simulink model "Model"  (R2025b)
settings: Solver=VariableStepAuto  StartTime=0.0  StopTime=1  RelTol=1e-3
values from neighbouring files (symbols this model uses):
  g = 9.81    [Main.m]
  i0 = 0.0    (= 0)    [Main.m]    (also in anonimousFunction.m)
  i_stable = u_stable / R    [Main.m]
  M = 0.058    [Model_parameters.m]
  m = 0.058    [Main.m]    (also in anonimousFunction.m)
  R = 3.9924    [Main.m]    (also in Model_parameters.m = 2.8304; Resistance_ident.m = fitobject.p1; anonimousFunction.m = 2)
  v0 = 0    [Main.m]    (also in anonimousFunction.m)
  v_stable = 0    [Main.m]
  x0 = 0.02    [Main.m]    (also in anonimousFunction.m)
  x_stable = 0.01    [Main.m]
undefined symbols (not defined in the file or in its folder): K
settings Model: Creator=janis  LastModifiedBy=Tim

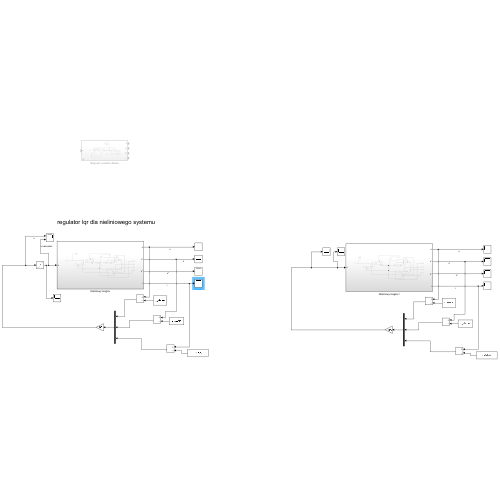
[thumbnail: Simulink's stored preview of the top-level diagram]
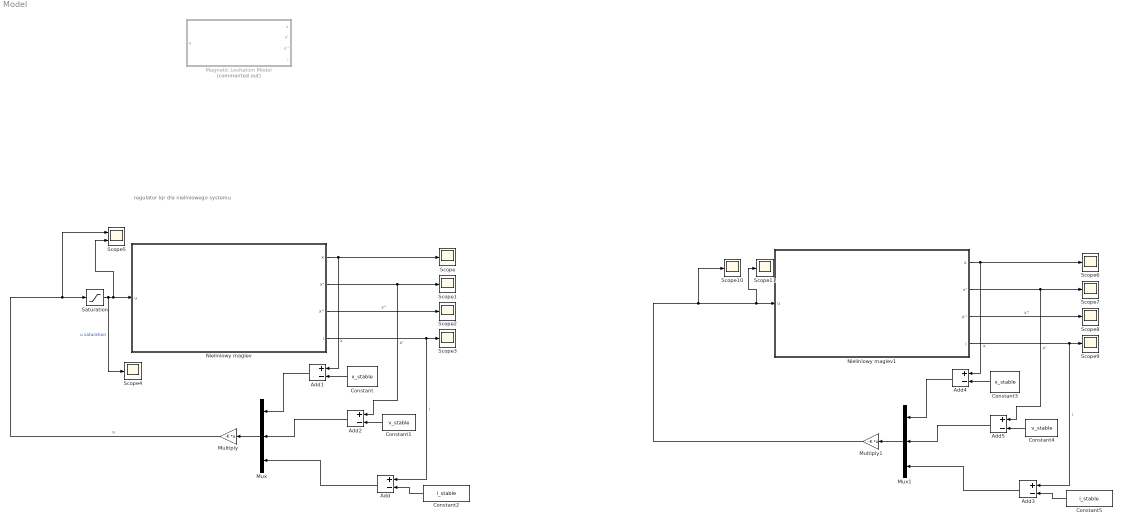
== system Model ==
  note: regulator lqr dla nieliniowego systemu
  Add{,1..5} (6 alike) : Sum  Inputs=+-
  Constant : Constant  Value=x_stable
  Constant1 : Constant  Value=v_stable
  Constant2 : Constant  Value=i_stable
  Constant3 : Constant  Value=x_stable
  Constant4 : Constant  Value=v_stable
  Constant5 : Constant  Value=i_stable
  Magnetic Levitation Model : Subsystem  Commented=on
  Multiply : Gain  Gain=-K  Multiplication=Matrix(K*u)
  Multiply1 : Gain  Gain=-K  Multiplication=Matrix(K*u)
  Mux : Mux  Inputs=3
  Mux1 : Mux  Inputs=3
  Nieliniowy maglev : Subsystem
  Nieliniowy maglev1 : Subsystem
  Saturation : Saturate  UpperLimit=11.3  LowerLimit=0
  Scope{,1..4,6..11} (11 alike) : Scope
      Scope settings: ActiveDisplayYMinimum=0.0081937181493075  ActiveDisplayYMaximum=0.026682726345841533  YLabel=x [m]
      Scope1 settings: ActiveDisplayYMinimum=-0.32675858583001738  ActiveDisplayYMaximum=0.19457434048931541  YLabel=x' [m/s]
      Scope10 settings: ActiveDisplayYMinimum=-8.0131796633081951  ActiveDisplayYMaximum=95.659493328647159  DataLoggingVariableName=ScopeData6
      Scope11 settings: ActiveDisplayYMinimum=-8.0131796633081951  ActiveDisplayYMaximum=95.659493328647159  DataLoggingVariableName=ScopeData7
      Scope2 settings: ActiveDisplayYMinimum=-15.369653428194885  ActiveDisplayYMaximum=12.607739269799431  YLabel=x'' [m/s^2]  DataLoggingVariableName=ScopeData2
      Scope3 settings: ActiveDisplayYMinimum=-0.53487282312330309  ActiveDisplayYMaximum=3.0849573402562789  YLabel=i [A]  DataLoggingVariableName=ScopeData3
      Scope4 settings: ActiveDisplayYMinimum=-0.37305316249219622  ActiveDisplayYMaximum=12.523736873656135  YLabel=u  DataLoggingVariableName=ScopeData4
      Scope6 settings: ActiveDisplayYMinimum=0.010968481395608059  ActiveDisplayYMaximum=0.021090683701156816  DataLoggingVariableName=ScopeData8
      Scope7 settings: ActiveDisplayYMinimum=-0.19832990389063207  ActiveDisplayYMaximum=0.16245757916094666  DataLoggingVariableName=ScopeData9
      Scope8 settings: ActiveDisplayYMinimum=-1  ActiveDisplayYMaximum=1  DataLoggingVariableName=ScopeData10
      Scope9 settings: ActiveDisplayYMinimum=-0.3151279377575355  ActiveDisplayYMaximum=2.83615143981782  DataLoggingVariableName=ScopeData11
  Scope5 : Scope  NumInputPorts=2
      settings: ActiveDisplayYMinimum=-56.44177745177619  ActiveDisplayYMaximum=512.64296076233984  DataLoggingVariableName=ScopeData5
  wires:
  Nieliniowy maglev/1(x) -> Scope/1, Add1/1  "x"
  Nieliniowy maglev/2(x') -> Add2/1, Scope1/1  "x'"
  Nieliniowy maglev/3(x'') -> Scope2/1  "x''"
  Nieliniowy maglev/4(i) -> Add/1, Scope3/1  "i"
  Constant2/1 -> Add/2
  Constant/1 -> Add1/2
  Constant1/1 -> Add2/2
  Mux/1 -> Multiply/1
  Add1/1 -> Mux/1
  Add2/1 -> Mux/2
  Multiply/1 -> Scope5/1, Saturation/1  "u"
  Add/1 -> Mux/3
  Saturation/1 -> Scope4/1, Scope5/2, Nieliniowy maglev/1(u)  "u saturation"
  Add3/1 -> Mux1/3
  Add4/1 -> Mux1/1
  Mux1/1 -> Multiply1/1
  Add5/1 -> Mux1/2
  Multiply1/1 -> Scope11/1, Nieliniowy maglev1/1(u), Scope10/1
  Nieliniowy maglev1/1(x) -> Scope6/1, Add4/1  "x"
  Constant3/1 -> Add4/2
  Nieliniowy maglev1/4(i) -> Add3/1, Scope9/1  "i"
  Nieliniowy maglev1/3(x'') -> Scope8/1  "x''"
  Nieliniowy maglev1/2(x') -> Add5/1, Scope7/1  "x'"
  Constant5/1 -> Add3/2
  Constant4/1 -> Add5/2

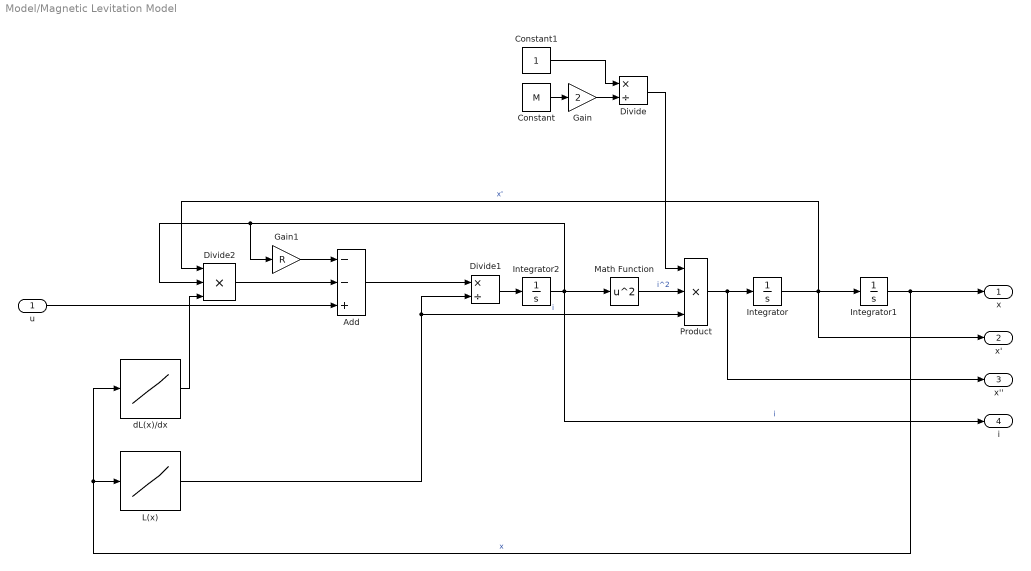
== system Model/Magnetic Levitation Model ==
  u : Inport
  Add : Sum  Inputs=--+
  Constant : Constant  Value=M
  Constant1 : Constant
  Divide : Product  Inputs=*/
  Divide1 : Product  Inputs=*/
  Divide2 : Product  Inputs=***
  Gain : Gain  Gain=2
  Gain1 : Gain  Gain=R
  Integrator : Integrator
  Integrator1 : Integrator
  Integrator2 : Integrator
  L(x) : Lookup_n-D  NumberOfTableDimensions=1  BreakpointsForDimension1=[-1:1]  Table=[-1:1]  InternalRulePriority=Speed  RndMeth=Simplest
  Math Function : Math  Operator=square
  Product : Product  Inputs=3
  dL(x)/dx : Lookup_n-D  NumberOfTableDimensions=1  BreakpointsForDimension1=[-1:1]  Table=[-1:1]  InternalRulePriority=Speed  RndMeth=Simplest
  x : Outport
  x' : Outport  Port=2
  x'' : Outport  Port=3
  i : Outport  Port=4
  wires:
  Gain1/1 -> Add/1
  L(x)/1 -> Divide1/2, Product/3  "i"
  Gain/1 -> Divide/2
  Divide2/1 -> Add/2
  Constant/1 -> Gain/1
  Integrator2/1 -> i/1, Gain1/1, Divide2/2, Math Function/1  "i"
  Integrator/1 -> x'/1, Divide2/1, Integrator1/1  "x'"
  Add/1 -> Divide1/1
  Integrator1/1 -> x/1, dL(x)/dx/1, L(x)/1  "x"
  Constant1/1 -> Divide/1
  Product/1 -> x''/1, Integrator/1
  Divide/1 -> Product/1
  Divide1/1 -> Integrator2/1
  dL(x)/dx/1 -> Divide2/3
  Math Function/1 -> Product/2  "i^2"
  u/1 -> Add/3

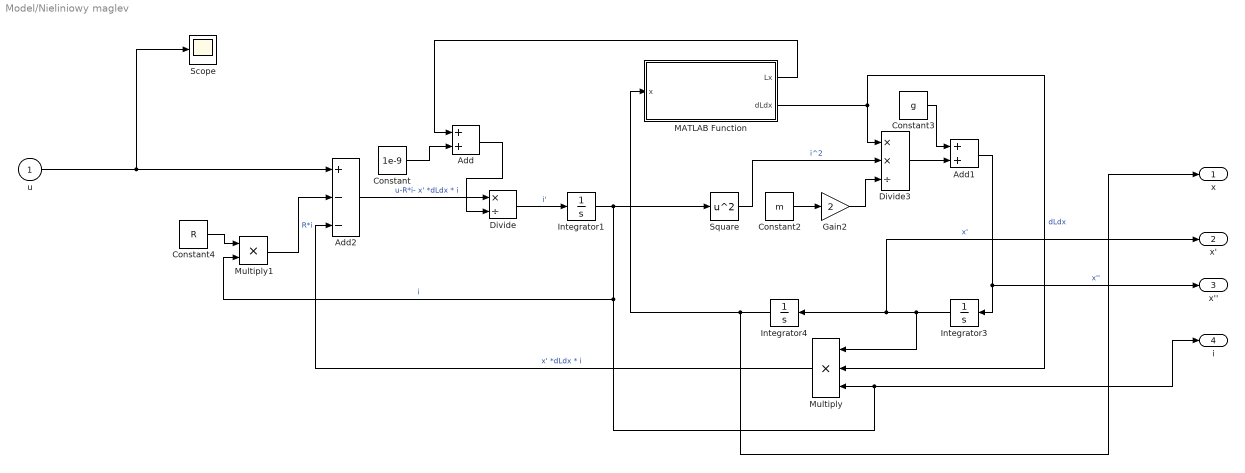
== system Model/Nieliniowy maglev ==
  u : Inport
  Add : Sum
  Add1 : Sum
  Add2 : Sum  Inputs=+--
  Constant : Constant  Value=1e-9
  Constant2 : Constant  Value=m
  Constant3 : Constant  Value=g
  Constant4 : Constant  Value=R
  Divide : Product  Inputs=*/
  Divide3 : Product  Inputs=**/
  Gain2 : Gain  Gain=2
  Integrator1 : Integrator  InitialCondition=i0
  Integrator3 : Integrator  InitialCondition=v0
  Integrator4 : Integrator  InitialCondition=x0
  MATLAB Function : MATLAB Function  TreatAsAtomicUnit=on
  Multiply : Product  Inputs=***
  Multiply1 : Product  Inputs=**
  Scope : Scope
      settings: ActiveDisplayYMinimum=-1  ActiveDisplayYMaximum=1  DataLoggingVariableName=ScopeData12
  Square : Math  Operator=square
  x : Outport
  x' : Outport  Port=2
  x'' : Outport  Port=3
  i : Outport  Port=4
  wires:
  Integrator3/1 -> Multiply/1, x'/1, Integrator4/1  "x'"
  Constant3/1 -> Add1/1
  MATLAB Function/2(dLdx) -> Divide3/1, Multiply/2  "dLdx"
  Add2/1 -> Divide/1  "u-R*i- x' *dLdx * i"
  Constant2/1 -> Gain2/1
  Integrator4/1 -> x/1, MATLAB Function/1(x)
  Gain2/1 -> Divide3/3
  Add/1 -> Divide/2
  Integrator1/1 -> i/1, Multiply/3, Multiply1/2, Square/1  "i"
  MATLAB Function/1(Lx) -> Add/1
  Divide/1 -> Integrator1/1  "i'"
  Constant/1 -> Add/2
  Add1/1 -> x''/1, Integrator3/1  "x''"
  Square/1 -> Divide3/2  "i^2"
  Divide3/1 -> Add1/2
  Multiply1/1 -> Add2/2  "R*i"
  Multiply/1 -> Add2/3  "x' *dLdx * i"
  u/1 -> Scope/1, Add2/1
  Constant4/1 -> Multiply1/1

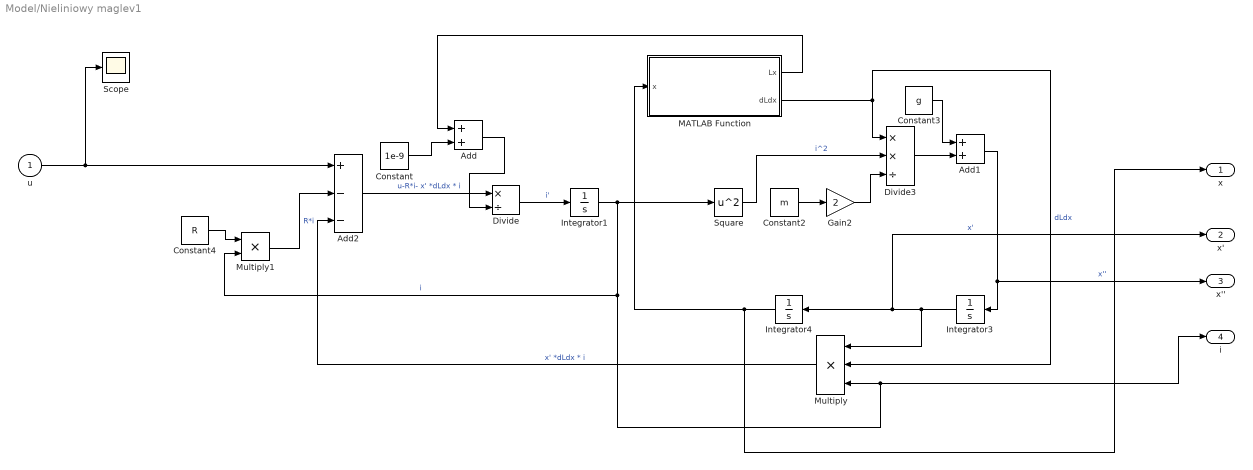
== system Model/Nieliniowy maglev1 ==
  u : Inport
  Add : Sum
  Add1 : Sum
  Add2 : Sum  Inputs=+--
  Constant : Constant  Value=1e-9
  Constant2 : Constant  Value=m
  Constant3 : Constant  Value=g
  Constant4 : Constant  Value=R
  Divide : Product  Inputs=*/
  Divide3 : Product  Inputs=**/
  Gain2 : Gain  Gain=2
  Integrator1 : Integrator  InitialCondition=i0
  Integrator3 : Integrator  InitialCondition=v0
  Integrator4 : Integrator  InitialCondition=x0
  MATLAB Function : MATLAB Function  TreatAsAtomicUnit=on
  Multiply : Product  Inputs=***
  Multiply1 : Product  Inputs=**
  Scope : Scope
      settings: ActiveDisplayYMinimum=-1  ActiveDisplayYMaximum=1  DataLoggingVariableName=ScopeData13
  Square : Math  Operator=square
  x : Outport
  x' : Outport  Port=2
  x'' : Outport  Port=3
  i : Outport  Port=4
  wires:
  Integrator3/1 -> Multiply/1, x'/1, Integrator4/1  "x'"
  Constant3/1 -> Add1/1
  MATLAB Function/2(dLdx) -> Divide3/1, Multiply/2  "dLdx"
  Add2/1 -> Divide/1  "u-R*i- x' *dLdx * i"
  Constant2/1 -> Gain2/1
  Integrator4/1 -> x/1, MATLAB Function/1(x)
  Gain2/1 -> Divide3/3
  Add/1 -> Divide/2
  Integrator1/1 -> i/1, Multiply/3, Multiply1/2, Square/1  "i"
  MATLAB Function/1(Lx) -> Add/1
  Divide/1 -> Integrator1/1  "i'"
  Constant/1 -> Add/2
  Add1/1 -> x''/1, Integrator3/1  "x''"
  Square/1 -> Divide3/2  "i^2"
  Divide3/1 -> Add1/2
  Multiply1/1 -> Add2/2  "R*i"
  Multiply/1 -> Add2/3  "x' *dLdx * i"
  u/1 -> Scope/1, Add2/1
  Constant4/1 -> Multiply1/1

== matlab function Model/Nieliniowy maglev/MATLAB Function ==
  data: x input; Lx output; dLdx output
function [Lx, dLdx] = Maglev_Inductance(x)
a = 0.0271;
b = -311.9855;
c = 0.1140;
d = -3.5209;

% Funkcja L(x)
Lx = a*exp(b*x) + c*exp(d*x);

% Pochodna dL/dx(x)
dLdx = a*b*exp(b*x) + c*d*exp(d*x);
end

== matlab function Model/Nieliniowy maglev1/MATLAB Function ==
  data: x input; Lx output; dLdx output
function [Lx, dLdx] = Maglev_Inductance(x)
a = 0.0271;
b = -311.9855;
c = 0.1140;
d = -3.5209;

% Funkcja L(x)
Lx = a*exp(b*x) + c*exp(d*x);

% Pochodna dL/dx(x)
dLdx = a*b*exp(b*x) + c*d*exp(d*x);
end
